simulink model "MPConFCC"  (R2016a)
settings: Solver=VariableStepAuto  StartTime=0.0  StopTime=20  RelTol=1e-3
values from neighbouring files (symbols this model uses):
  C = Cbar*C_new    [MPCmain.m]    (also in Params.m)
  m = 6    [MPCmain.m]    (also in Params.m)
  p = 12    [MPCmain.m]    (also in Params.m)
  P00 = 100*[0.001 0.003 0.003 0.003 ... (first row only)    [Params.m]
  Q = 0.1*diag([1 1 1])    [Params.m]
  Qu = eye(2)    [MPCmain.m]    (also in Params.m)
  Qy = diag([10000000 10000000 1])    [MPCmain.m]    (also in Params.m)
  R = eye(3,3)*0.01    [Params.m]
  Ref = [0.03 0.25 375]'    [MPCmain.m]    (also in Params.m)
  X00 = X0    [Params.m]
undefined symbols (not defined in the file or in its folder): A, B, Ts
settings Model: Creator=hp  LastModifiedBy=hp

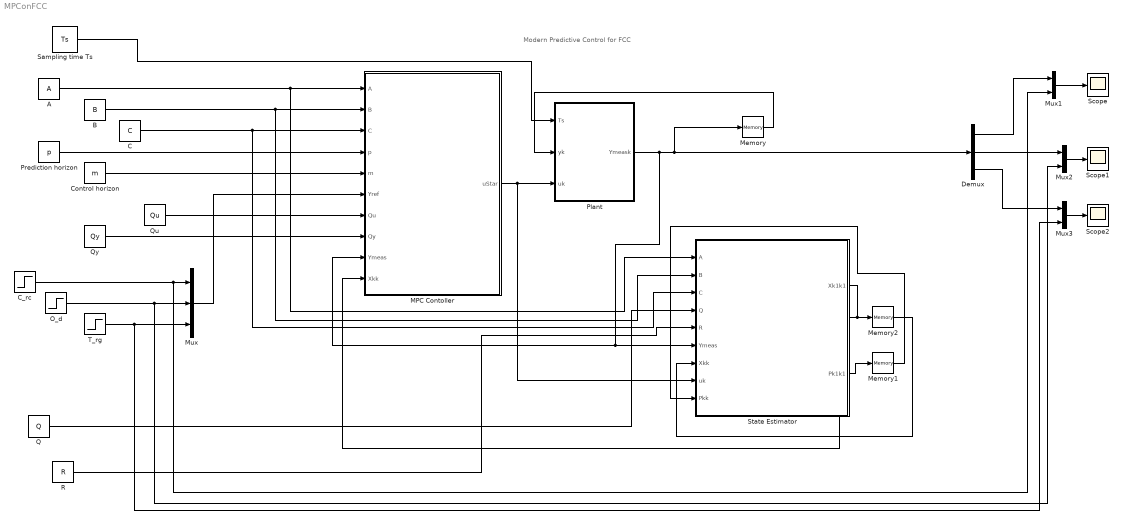
== system MPConFCC ==
  note: Modern Predictive Control for FCC
  A : Constant  Value=A  VectorParams1D=off
  B : Constant  Value=B  VectorParams1D=off
  C : Constant  Value=C  VectorParams1D=off
  C_rc : Step  Time=0  After=Ref(1)  SampleTime=Ts
  Control horizon : Constant  Value=m
  Demux : Demux  Outputs=3
  MPC Contoller : MATLAB Function  TreatAsAtomicUnit=on
  Memory : Memory  X0=C*X00  InheritSampleTime=on
  Memory1 : Memory  X0=P00
  Memory2 : Memory  X0=X00
  Mux : Mux  Inputs=3
  Mux1 : Mux  Inputs=2
  Mux2 : Mux  Inputs=2
  Mux3 : Mux  Inputs=2
  O_d : Step  Time=0  After=Ref(2)  SampleTime=Ts
  Plant : MATLAB Function  TreatAsAtomicUnit=on
  Prediction horizon : Constant  Value=p
  Q : Constant  Value=Q  VectorParams1D=off
  Qu : Constant  Value=Qu  VectorParams1D=off
  Qy : Constant  Value=Qy  VectorParams1D=off
  R : Constant  Value=R  VectorParams1D=off
  Sampling time Ts : Constant  Value=Ts
  Scope : Scope
  Scope1 : Scope
  Scope2 : Scope
  State Estimator : MATLAB Function  TreatAsAtomicUnit=on
  T_rg : Step  After=Ref(3)  SampleTime=Ts
  wires:
  Sampling time Ts/1 -> Plant/1(Ts)
  MPC Contoller/1(uStar) -> State Estimator/8(uk), Plant/3(uk)
  A/1 -> State Estimator/1(A), MPC Contoller/1(A)
  B/1 -> State Estimator/2(B), MPC Contoller/2(B)
  C/1 -> State Estimator/3(C), MPC Contoller/3(C)
  State Estimator/1(Xk1k1) -> MPC Contoller/10(Xkk), Memory2/1
  Q/1 -> State Estimator/4(Q)
  R/1 -> State Estimator/5(R)
  Prediction horizon/1 -> MPC Contoller/4(p)
  Control horizon/1 -> MPC Contoller/5(m)
  Mux/1 -> MPC Contoller/6(Yref)
  C_rc/1 -> Mux1/2, Mux/1
  O_d/1 -> Mux/2, Mux2/2
  T_rg/1 -> Mux/3, Mux3/2
  Memory/1 -> Plant/2(yk)
  Memory2/1 -> State Estimator/7(Xkk)
  State Estimator/2(Pk1k1) -> Memory1/1
  Memory1/1 -> State Estimator/9(Pkk)
  Demux/1 -> Mux1/1
  Demux/2 -> Mux2/1
  Demux/3 -> Mux3/1
  Mux3/1 -> Scope2/1
  Mux2/1 -> Scope1/1
  Qu/1 -> MPC Contoller/7(Qu)
  Qy/1 -> MPC Contoller/8(Qy)
  Plant/1(Ymeask) -> State Estimator/6(Ymeas), MPC Contoller/9(Ymeas), Demux/1, Memory/1
  Mux1/1 -> Scope/1

== matlab function MPConFCC/Plant ==
  data: Ts input; yk input; uk input; Ymeask output
function Ymeask = plant(Ts,yk,uk)

    tspan  = [0 Ts];              % [startTime endTime]
    fun=@(t,y)yrates(t,y,uk);
    [tout, yout]    = ode45(fun, tspan, yk, 0.00000001);
    Ymeask = (yout(end,:))';   % predicted estimated
end

== matlab function MPConFCC/MPC Contoller ==
  data: A input; uStar output; B input; C input; p input; m input; Yref input; Qu input; Qy input; Ymeas input; Xkk input
function uStar = inputPlanSim(A,B,C, p,m,Yref,Qu,Qy,Ymeas, Xkk)

%{
A,B,C  - State space model matrices
Xkk    - Current estimated state
Yref   - Reference measurement for the prediction horizon size Nxp 
N      - number of measurements
L      - number of inputs
p      - Prediction horizon
m      - control horizon
Qu     - input weights
Qy     - measurement weights
%}






%%
[n, L] = size(B);
[N,~]  = size(C);
H      = 0 ;
f      = 0 ; 

for i = 1:p
    CABj = CABhoriz(A,B,C,i,m);
    H = H + CABj'*Qy*CABj;
    f = f + Xkk'*(A^i)'*C'*Qy*CABj -Yref(:,i)'*Qy*CABj;
end

QuBlock = Qu;
for  b = 1:m-1
    QuBlock = blkdiag(QuBlock,Qu)
end
H = H+QuBlock; 
uStar = quadprog(H,f);
uStar = reshape(uStar,L,[]);
uStar = [uStar uStar(:,end)*ones(1,p-m)];
end

== matlab function MPConFCC/State Estimator ==
  data: A input; Xk1k1 output; B input; C input; Q input; R input; Ymeas input; Xkk input; uk input; Pkk input; Pk1k1 output
function [Xk1k1,Pk1k1] = KalmanFilter(A,B,C,Q,R,Ymeas,Xkk,uk,Pkk)

s     = size(Pkk);
    % Prediction
    Xk1k=A*Xkk+B*uk;
    Pk1k=A*Pkk*A'+Q;
     % Correction
    K=Pk1k*C'*inv(C*Pk1k*C'+R);        % Optimal Kalman gain
    Xk1k1=Xk1k+K*(Ymeas-C*Xk1k);
    
    Pk1k1=(eye(s)-K*C)*Pk1k;


end
